simulink model "doc_mtailbiting_wfeedback"  (R2014a)
settings: Solver=FixedStepDiscrete  StartTime=0.0  StopTime=100.0  RelTol=1e-3
PreLoadFcn:
  | blkLen = 10;
  | trellis = poly2trellis(3,[7 5],7);
  | mapStValues = [0 2 3 1];
libraries: commcnvcod2 x2, commrandsrc2 x1
settings Model: Creator=The MathWorks Inc.
settings DataIOCC: SignalLoggingSaveFormat=ModelDataLogs
settings OptimizationCC: ExpressionDepthLimit=2147483647  EfficientMapNaN2IntZero=off
settings DebuggingCC: UnderspecifiedInitializationDetection=Classic  FcnCallInpInsideContextMsg=UseLocalSettings  StateNameClashWarn=warning  StrictBusMsg=Warning
settings GRTTargetCC: CombineOutputUpdateFcns=off  GRTInterface=on

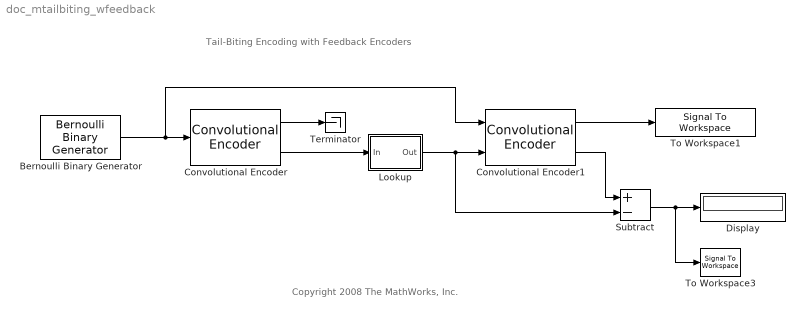
== system doc_mtailbiting_wfeedback ==
  note: Tail-Biting Encoding with Feedback Encoders
  note: Copyright 2008 The MathWorks, Inc.
  Bernoulli Binary Generator : commrandsrc2/Bernoulli Binary Generator  P=0.5  seed=61  Ts=0.1  frameBased=on  sampPerFrame=blkLen  orient=off  outDataType=boolean
  Convolutional Encoder : commcnvcod2/Convolutional Encoder  trellis=trellis  opMode=Truncated (reset every frame)  DelayedResetAction=off  hasIniStPort=off  hasFinStPort=on  usePuncVector=off  punctureVector=[1; 1; 0; 1; 0; 1]  reset=Unused parameter value
  Convolutional Encoder1 : commcnvcod2/Convolutional Encoder  trellis=trellis  opMode=Truncated (reset every frame)  DelayedResetAction=off  hasIniStPort=on  hasFinStPort=on  usePuncVector=off  punctureVector=[1; 1; 0; 1; 0; 1]  reset=Unused parameter value
  Display : Display
  Lookup : Subsystem  TreatAsAtomicUnit=on
  Subtract : Sum  Inputs=+-
  Terminator : Terminator
  To Workspace1 : SignalToWorkspace  VariableName=encoded_out
  To Workspace3 : SignalToWorkspace  VariableName=out
  wires:
  Subtract/1 -> Display/1, To Workspace3/1
  Convolutional Encoder1/2 -> Subtract/1
  Convolutional Encoder/1 -> Terminator/1
  Convolutional Encoder/2 -> Lookup/1(In)
  Lookup/1(Out) -> Convolutional Encoder1/2, Subtract/2
  Bernoulli Binary Generator/1 -> Convolutional Encoder/1, Convolutional Encoder1/1
  Convolutional Encoder1/1 -> To Workspace1/1

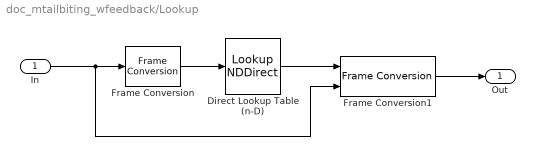
== system doc_mtailbiting_wfeedback/Lookup ==
  In : Inport
  Direct Lookup Table (n-D) : LookupNDDirect  NumberOfTableDimensions=1  Table=mapStValues  DiagnosticForOutOfRangeInput=Error
  Frame Conversion : FrameConversion  OutFrame=Sample-based
  Frame Conversion1 : FrameConversion  InheritSamplingMode=on  OutFrame=Sample-based
  Out : Outport
  wires:
  In/1 -> Frame Conversion/1, Frame Conversion1/2
  Frame Conversion/1 -> Direct Lookup Table (n-D)/1
  Direct Lookup Table (n-D)/1 -> Frame Conversion1/1
  Frame Conversion1/1 -> Out/1
